simulink model "secorderpid2nd_add_filters"  (R2020a)
settings: Solver=ode23  StartTime=0.0  StopTime=30  FixedStep=1e-3  MaxStep=5e-4  RelTol=5e-4
values from neighbouring files (symbols this model uses):
  b = [1 0]    [Exemple_2_disertacao.mat]    (also in Lpid.m = j*w(a); example_result_gasearch_nelson_com_PID.mat = [0 0 1 1])
  C = [1  -0.9999; -0.9999  1]    [Exemple_2_disertacao.mat]    (also in example2MG.mat = [0.5 0 0 0 0 0 0 0 0 0 0 0 ... (16 elements, 4x4)]; example_result_gasearch_nelson_com_PID.mat = [0.5 0 -0.5 0 0 0 0 0 -0.5 0 0.5 0 ... (16 elements, 4x4)]; wingcons.mat = [7.66  2.45  2.1; 0.23  1.04  0.223; 0.6  0.756  0.658])
  d = [1 0]    [Exemple_2_disertacao.mat]    (also in Exemple_6_disertacao.mat; example2MG.mat = [1 6 15 18 10]; example_result_gasearch_nelson_com_PID.mat = [0 0 1 1])
  dx0 = [0 0]    [Exemple_2_disertacao.mat]    (also in Exemple_6_disertacao.mat; example2MG.mat = [0 0 0 0])
  K = [2.5 -1 0 0 0 0 0 0 0 0 0 0 ... (2500 elements, 50x50)]    [Belloti_N50.mat]    (also in Exemple_2_disertacao.mat = [3  -2; -2  3]; Exemple_6_disertacao.mat = [3  -2; -2  3]; example2MG.mat = [5 -5 0 0 -5 10 -5 0 0 -5 10 -5 ... (16 elements, 4x4)]; example_result_gasearch_nelson_com_PID.mat = [200 0 -100 0 0 200 0 -100 -100 0 150 -50 ... (16 elements, )
  M = [4 0 0 0 0 0 0 0 0 0 0 0 ... (2500 elements, 50x50)]    [Belloti_N50.mat]    (also in Exemple_2_disertacao.mat = [1  0; 0  1]; Exemple_6_disertacao.mat = [1  0; 0  1]; example2MG.mat = [1 0 0 0 0 1 0 0 0 0 1 0 ... (16 elements, 4x4)]; example_result_gasearch_nelson_com_PID.mat = [1 0 0 0 0 1 0 0 0 0 1 0 ... (16 elements, 4x4)])
  tau = 0.1    [Belloti_N50.mat]    (also in Exemple_2_disertacao.mat = 0.5; Exemple_6_disertacao.mat = 0.5; example_result_gasearch_nelson_com_PID.mat = 0.05)
  x0 = [1 0 0 0 0 0 0 0 0 0 0 0 ... (50 elements, 1x50)]    [Belloti_N50.mat]    (also in Exemple_2_disertacao.mat = [0 0]; Exemple_6_disertacao.mat = [0 0]; example2MG.mat = [0 0 0 0]; example_result_gasearch_nelson_com_PID.mat = [1 0 0 0])
settings Model: Creator=Jose  LastModifiedBy=jhona
settings DataIOCC: LimitDataPoints=on  SaveFormat=Array  SignalLoggingSaveFormat=ModelDataLogs  ReturnWorkspaceOutputs=off
settings OptimizationCC: BlockReduction=off  BooleanDataType=off  ExpressionDepthLimit=2147483647  EfficientMapNaN2IntZero=off  LifeSpan=inf
settings DebuggingCC: SaveWithParameterizedLinksMsg=none  UnderspecifiedInitializationDetection=Classic  MergeDetectMultiDrivingBlocksExec=none  SignalResolutionControl=TryResolveAllWithWarning  MultiTaskDSMMsg=warning  MultiTaskCondExecSysMsg=none  StateNameClashWarn=warning  SFUnexpectedBacktrackingDiag=warning  SFNoUnconditionalDefaultTransitionDiag=warning  SFExecutionAtInitializationDiag=none  ArithmeticOperatorsInVariantConditions=warning
settings HardwareCC: ProdBitPerPointer=32  ProdBitPerSizeT=32  ProdBitPerPtrDiffT=32  ProdLargestAtomicFloat=None  ProdIntDivRoundTo=Undefined  ProdEndianess=Unspecified  ProdWordSize=32  ProdHWDeviceType=32-bit Generic  TargetBitPerPointer=64  TargetBitPerSizeT=64  TargetBitPerPtrDiffT=64  TargetLongLongMode=on  TargetIntDivRoundTo=Zero  TargetEndianess=LittleEndian  TargetWordSize=64  TargetHWDeviceType=MATLAB Host  ProdEqTarget=off
settings ModelReferenceCC: PropagateSignalLabelsOutOfModel=off
settings SFSimCC: SimUseLocalCustomCode=off  CustomCodeUndefinedFunction=UseInterfaceOnly
settings RTWCC: RTWUseLocalCustomCode=off
settings CodeAppCC: MaxIdLength=128  StateflowObjectComments=on
settings GRTTargetCC: TargetLangStandard=C89/C90 (ANSI)  CombineOutputUpdateFcns=off  GRTInterface=on
settings ConfigComp: CovMetricSettings=dw  CovHtmlReporting=on  CovSaveCumulativeToWorkspaceVar=on  CovSaveSingleToWorkspaceVar=on  CovExternalEMLEnable=off

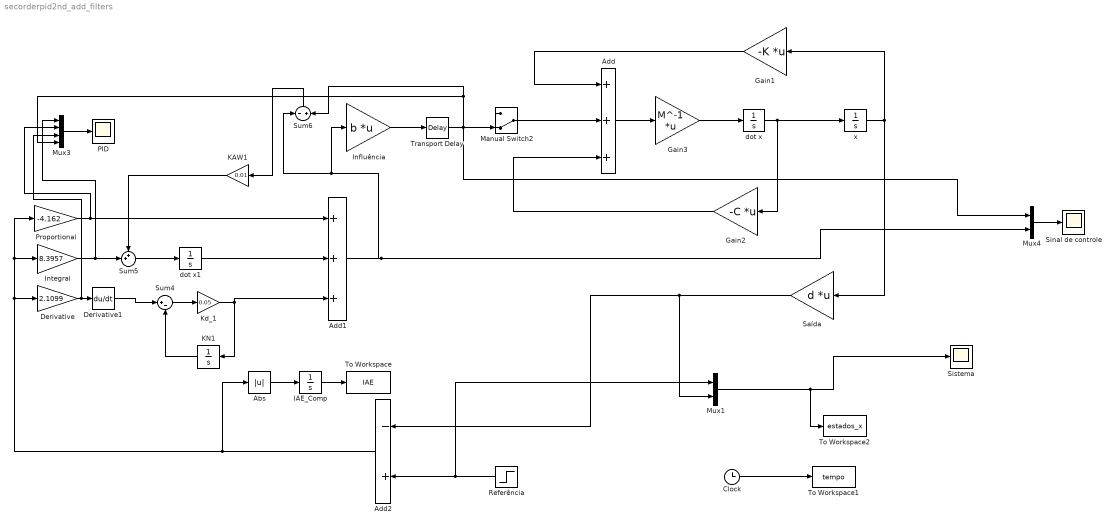
== system secorderpid2nd_add_filters ==
  Abs : Abs
  Add : Sum  Inputs=+++
  Add1 : Sum  Inputs=+++
  Add2 : Sum  Inputs=-+
  Clock : Clock
  Derivative : Gain  Gain=2.1099
  Derivative1 : Derivative  CoefficientInTFapproximation=100
  Gain1 : Gain  Gain=-K  Multiplication=Matrix(K*u)
  Gain2 : Gain  Gain=-C  Multiplication=Matrix(K*u)
  Gain3 : Gain  Gain=M^-1  Multiplication=Matrix(K*u)
  IAE_Comp : Integrator
  Influência : Gain  Gain=b  Multiplication=Matrix(K*u)
  Integral : Gain  Gain=8.3957
  KAW1 : Gain  Gain=0.01
  KN1 : Integrator
  Kd_1 : Gain  Gain=0.05
  Manual Switch2 : ManualSwitch  CurrentSetting=0
  Mux1 : Mux  Inputs=2
  Mux3 : Mux
  Mux4 : Mux  Inputs=2
  PID : Scope
  Proportional : Gain  Gain=-4.162
  Referência : Step  Time=0  SampleTime=0
  Saída : Gain  Gain=d  Multiplication=Matrix(K*u)
  Sinal de controle : Scope
  Sistema : Scope
  Sum4 : Sum  Inputs=|+-
  Sum5 : Sum  Inputs=++|
  Sum6 : Sum  Inputs=-|+
  To Workspace : ToWorkspace  VariableName=IAE  SampleTime=-1
  To Workspace1 : ToWorkspace  VariableName=tempo  SampleTime=-1
  To Workspace2 : ToWorkspace  VariableName=estados_x  SampleTime=-1
  Transport Delay : TransportDelay  DelayTime=tau  BufferSize=2048
  dot x : Integrator  InitialCondition=dx0
  dot x1 : Integrator
  x : Integrator  InitialCondition=x0
  wires:
  Gain1/1 -> Add/1
  Add/1 -> Gain3/1
  Gain3/1 -> dot x/1
  x/1 -> Saída/1, Gain1/1
  dot x/1 -> Gain2/1, x/1
  Gain2/1 -> Add/3
  Influência/1 -> Transport Delay/1
  Manual Switch2/1 -> Add/2
  Proportional/1 -> Mux3/2, Add1/1
  dot x1/1 -> Add1/2
  Derivative/1 -> Mux3/3, Derivative1/1
  Referência/1 -> Mux1/1, Add2/2
  Add1/1 -> Mux4/2, Influência/1, Sum6/1
  Add2/1 -> Abs/1, Proportional/1, Integral/1, Derivative/1
  Abs/1 -> IAE_Comp/1
  IAE_Comp/1 -> To Workspace/1
  Clock/1 -> To Workspace1/1
  Mux1/1 -> To Workspace2/1, Sistema/1
  Saída/1 -> Add2/1, Mux1/2
  Transport Delay/1 -> Mux3/4, Sum6/2, Mux4/1, Manual Switch2/2
  Kd_1/1 -> KN1/1, Add1/3
  Sum4/1 -> Kd_1/1
  KN1/1 -> Sum4/2
  Derivative1/1 -> Sum4/1
  Integral/1 -> Mux3/1, Sum5/2
  Sum5/1 -> dot x1/1
  KAW1/1 -> Sum5/1
  Sum6/1 -> KAW1/1
  Mux4/1 -> Sinal de controle/1
  Mux3/1 -> PID/1
